simulink library "Library_DataProcessing_v1_1"  (R2021b)
settings: Solver=VariableStepAuto  StartTime=0.0  StopTime=10.0  RelTol=1e-3
libraries: simulink x6, hdlsllib x2
settings Model: Creator=SidharthUrbanMobilit  LastModifiedBy=SiddharthUrbanMobili

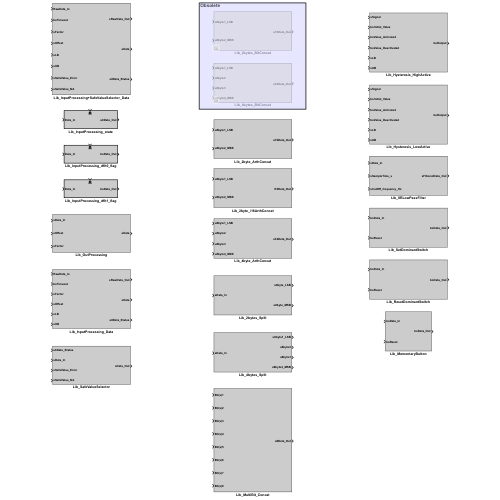
[thumbnail: Simulink's stored preview of the top-level diagram]
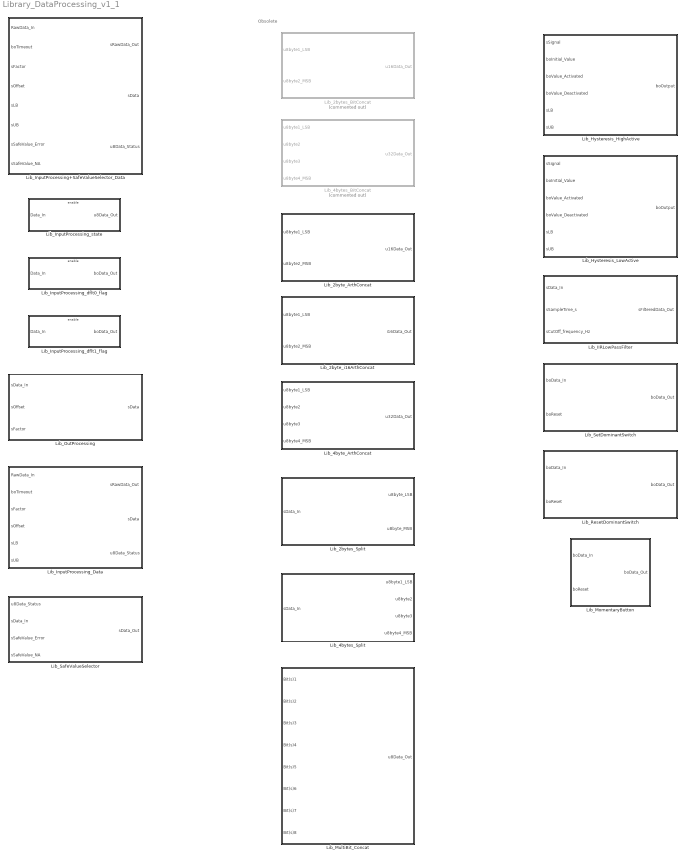
== system Library_DataProcessing_v1_1 ==
  note: Obsolete
  Lib_2byte_ArthConcat : Subsystem
      settings: RTWFcnNameOpts=Use subsystem name  RTWFileNameOpts=Use subsystem name
  Lib_2byte_i16ArthConcat : Subsystem
      settings: RTWFcnNameOpts=Use subsystem name  RTWFileNameOpts=Use subsystem name
  Lib_2bytes_BitConcat : Subsystem  Commented=on
  Lib_2bytes_Split : Subsystem
  Lib_4byte_ArthConcat : Subsystem
      settings: RTWFcnNameOpts=Use subsystem name  RTWFileNameOpts=Use subsystem name
  Lib_4bytes_BitConcat : Subsystem  Commented=on
  Lib_4bytes_Split : Subsystem
  Lib_Hysteresis_HighActive : Subsystem
  Lib_Hysteresis_LowActive : Subsystem
  Lib_IIRLowPassFilter : Subsystem
  Lib_InputProcessing+SafeValueSelector_Data : Subsystem
  Lib_InputProcessing_Data : Subsystem
  Lib_InputProcessing_dflt0_flag : Subsystem
  Lib_InputProcessing_dflt1_flag : Subsystem
  Lib_InputProcessing_state : Subsystem
  Lib_MomentaryButton : Subsystem
  Lib_MultiBit_Concat : Subsystem
      settings: RTWFcnNameOpts=Use subsystem name  RTWFileNameOpts=Use subsystem name
  Lib_OutProcessing : Subsystem
  Lib_ResetDominantSwitch : Subsystem
  Lib_SafeValueSelector : Subsystem
  Lib_SetDominantSwitch : Subsystem

== system Library_DataProcessing_v1_1/Lib_2byte_ArthConcat ==
  u8byte1_LSB : Inport  OutDataTypeStr=uint8
  u8byte2_MSB : Inport  Port=2  OutDataTypeStr=uint8
  Add : Sum  OutDataTypeStr=uint16  RndMeth=Nearest
  Data Type Conversion : DataTypeConversion  OutDataTypeStr=uint16
  Shift Arithmetic : ArithShift  BitShiftNumber=8  BitShiftDirection=Left
  u16Data_Out : Outport
  wires:
  u8byte2_MSB/1 -> Data Type Conversion/1
  Shift Arithmetic/1 -> Add/1
  u8byte1_LSB/1 -> Add/2
  Add/1 -> u16Data_Out/1
  Data Type Conversion/1 -> Shift Arithmetic/1

== system Library_DataProcessing_v1_1/Lib_2byte_i16ArthConcat ==
  u8byte1_LSB : Inport  OutDataTypeStr=uint8
  u8byte2_MSB : Inport  Port=2  OutDataTypeStr=uint8
  Add : Sum  OutDataTypeStr=int16  RndMeth=Nearest
  Data Type Conversion : DataTypeConversion  OutDataTypeStr=int16
  Shift Arithmetic : ArithShift  BitShiftNumber=8  BitShiftDirection=Left
  i16Data_Out : Outport
  wires:
  Data Type Conversion/1 -> Shift Arithmetic/1
  Add/1 -> i16Data_Out/1
  u8byte1_LSB/1 -> Add/2
  Shift Arithmetic/1 -> Add/1
  u8byte2_MSB/1 -> Data Type Conversion/1

== system Library_DataProcessing_v1_1/Lib_2bytes_BitConcat ==
  u8byte1_LSB : Inport  OutDataTypeStr=uint8
  u8byte2_MSB : Inport  Port=2  OutDataTypeStr=uint8
  Bit Concat : hdlsllib/Logic and Bit Operations/Bit Concat  numInputs=2
  Data Type Conversion : DataTypeConversion  OutDataTypeStr=uint16  RndMeth=Nearest
  u16Data_Out : Outport  OutDataTypeStr=uint16
  wires:
  Bit Concat/1 -> Data Type Conversion/1
  Data Type Conversion/1 -> u16Data_Out/1
  u8byte2_MSB/1 -> Bit Concat/1
  u8byte1_LSB/1 -> Bit Concat/2

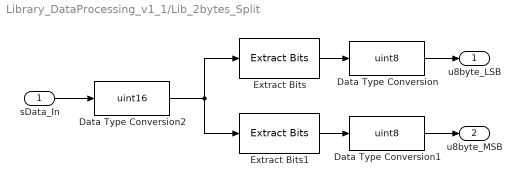
== system Library_DataProcessing_v1_1/Lib_2bytes_Split ==
  sData_In : Inport  OutDataTypeStr=single
  Data Type Conversion : DataTypeConversion  OutDataTypeStr=uint8  RndMeth=Nearest
  Data Type Conversion1 : DataTypeConversion  OutDataTypeStr=uint8  RndMeth=Nearest
  Data Type Conversion2 : DataTypeConversion  OutDataTypeStr=uint16  RndMeth=Nearest
  Extract Bits : simulink/Logic and Bit Operations/Extract Bits  bitsToExtract=Range of bits  numBits=8  bitIdxRange=[0 7]  outScalingMode=Treat bit field as an integer
  Extract Bits1 : simulink/Logic and Bit Operations/Extract Bits  bitsToExtract=Range of bits  numBits=8  bitIdxRange=[8 15]  outScalingMode=Treat bit field as an integer
  u8byte_LSB : Outport
  u8byte_MSB : Outport  Port=2
  wires:
  Extract Bits/1 -> Data Type Conversion/1
  Extract Bits1/1 -> Data Type Conversion1/1
  Data Type Conversion/1 -> u8byte_LSB/1
  Data Type Conversion1/1 -> u8byte_MSB/1
  sData_In/1 -> Data Type Conversion2/1
  Data Type Conversion2/1 -> Extract Bits/1, Extract Bits1/1

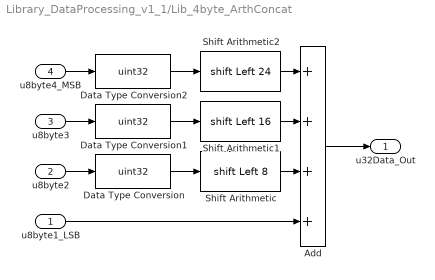
== system Library_DataProcessing_v1_1/Lib_4byte_ArthConcat ==
  u8byte1_LSB : Inport  OutDataTypeStr=uint8
  u8byte2 : Inport  Port=2  OutDataTypeStr=uint8
  u8byte3 : Inport  Port=3  OutDataTypeStr=uint8
  u8byte4_MSB : Inport  Port=4  OutDataTypeStr=uint8
  Add : Sum  Inputs=++++  OutDataTypeStr=uint32  RndMeth=Nearest
  Data Type Conversion : DataTypeConversion  OutDataTypeStr=uint32  RndMeth=Nearest
  Data Type Conversion1 : DataTypeConversion  OutDataTypeStr=uint32  RndMeth=Nearest
  Data Type Conversion2 : DataTypeConversion  OutDataTypeStr=uint32  RndMeth=Nearest
  Shift Arithmetic : ArithShift  BitShiftNumber=8  BitShiftDirection=Left
  Shift Arithmetic1 : ArithShift  BitShiftNumber=16  BitShiftDirection=Left
  Shift Arithmetic2 : ArithShift  BitShiftNumber=24  BitShiftDirection=Left
  u32Data_Out : Outport
  wires:
  Data Type Conversion/1 -> Shift Arithmetic/1
  Add/1 -> u32Data_Out/1
  u8byte2/1 -> Data Type Conversion/1
  Data Type Conversion1/1 -> Shift Arithmetic1/1
  u8byte3/1 -> Data Type Conversion1/1
  Data Type Conversion2/1 -> Shift Arithmetic2/1
  u8byte4_MSB/1 -> Data Type Conversion2/1
  Shift Arithmetic2/1 -> Add/1
  Shift Arithmetic1/1 -> Add/2
  Shift Arithmetic/1 -> Add/3
  u8byte1_LSB/1 -> Add/4

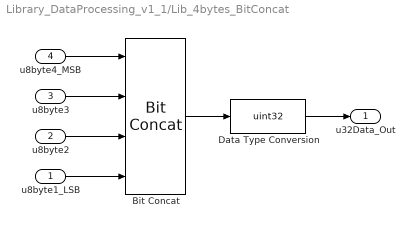
== system Library_DataProcessing_v1_1/Lib_4bytes_BitConcat ==
  u8byte1_LSB : Inport  OutDataTypeStr=uint8
  u8byte2 : Inport  Port=2  OutDataTypeStr=uint8
  u8byte3 : Inport  Port=3  OutDataTypeStr=uint8
  u8byte4_MSB : Inport  Port=4  OutDataTypeStr=uint8
  Bit Concat : hdlsllib/Logic and Bit Operations/Bit Concat  numInputs=4
  Data Type Conversion : DataTypeConversion  OutDataTypeStr=uint32  RndMeth=Nearest
  u32Data_Out : Outport  OutDataTypeStr=uint32
  wires:
  Data Type Conversion/1 -> u32Data_Out/1
  Bit Concat/1 -> Data Type Conversion/1
  u8byte4_MSB/1 -> Bit Concat/1
  u8byte3/1 -> Bit Concat/2
  u8byte2/1 -> Bit Concat/3
  u8byte1_LSB/1 -> Bit Concat/4

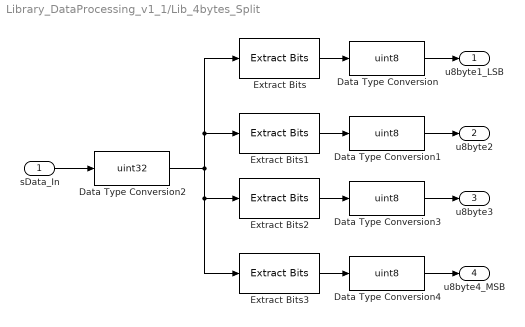
== system Library_DataProcessing_v1_1/Lib_4bytes_Split ==
  sData_In : Inport  OutDataTypeStr=single
  Data Type Conversion{,1,3..4} (4 alike) : DataTypeConversion  OutDataTypeStr=uint8  RndMeth=Nearest
  Data Type Conversion2 : DataTypeConversion  OutDataTypeStr=uint32  RndMeth=Nearest
  Extract Bits : simulink/Logic and Bit Operations/Extract Bits  bitsToExtract=Range of bits  numBits=8  bitIdxRange=[0 7]  outScalingMode=Treat bit field as an integer
  Extract Bits1 : simulink/Logic and Bit Operations/Extract Bits  bitsToExtract=Range of bits  numBits=8  bitIdxRange=[8 15]  outScalingMode=Treat bit field as an integer
  Extract Bits2 : simulink/Logic and Bit Operations/Extract Bits  bitsToExtract=Range of bits  numBits=8  bitIdxRange=[16 23]  outScalingMode=Treat bit field as an integer
  Extract Bits3 : simulink/Logic and Bit Operations/Extract Bits  bitsToExtract=Range of bits  numBits=8  bitIdxRange=[24 31]  outScalingMode=Treat bit field as an integer
  u8byte1_LSB : Outport
  u8byte2 : Outport  Port=2
  u8byte3 : Outport  Port=3
  u8byte4_MSB : Outport  Port=4
  wires:
  Data Type Conversion2/1 -> Extract Bits3/1, Extract Bits2/1, Extract Bits/1, Extract Bits1/1
  sData_In/1 -> Data Type Conversion2/1
  Data Type Conversion1/1 -> u8byte2/1
  Data Type Conversion/1 -> u8byte1_LSB/1
  Extract Bits1/1 -> Data Type Conversion1/1
  Extract Bits/1 -> Data Type Conversion/1
  Extract Bits2/1 -> Data Type Conversion3/1
  Extract Bits3/1 -> Data Type Conversion4/1
  Data Type Conversion3/1 -> u8byte3/1
  Data Type Conversion4/1 -> u8byte4_MSB/1

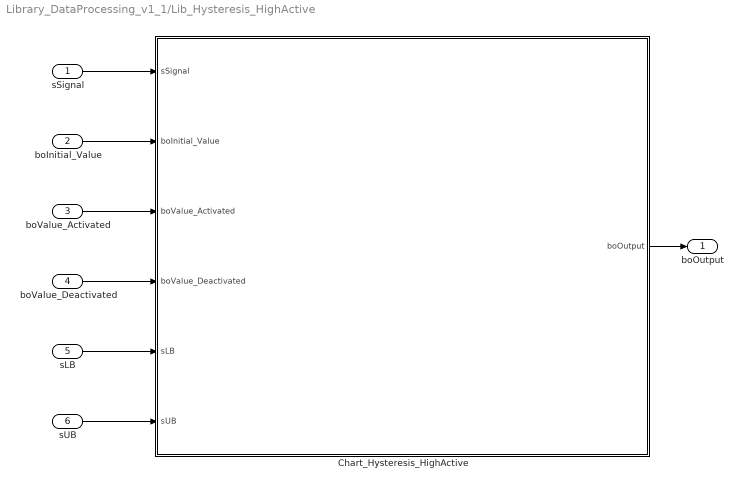
== system Library_DataProcessing_v1_1/Lib_Hysteresis_HighActive ==
  sSignal : Inport  OutDataTypeStr=single
  boInitial_Value : Inport  Port=2  OutDataTypeStr=boolean
  boValue_Activated : Inport  Port=3  OutDataTypeStr=boolean
  boValue_Deactivated : Inport  Port=4  OutDataTypeStr=boolean
  sLB : Inport  Port=5  OutDataTypeStr=single
  sUB : Inport  Port=6  OutDataTypeStr=single
  Chart_Hysteresis_HighActive : Stateflow chart  TreatAsAtomicUnit=on
  boOutput : Outport  OutDataTypeStr=boolean
  wires:
  boInitial_Value/1 -> Chart_Hysteresis_HighActive/2(boInitial_Value)
  boValue_Activated/1 -> Chart_Hysteresis_HighActive/3(boValue_Activated)
  sLB/1 -> Chart_Hysteresis_HighActive/5(sLB)
  sUB/1 -> Chart_Hysteresis_HighActive/6(sUB)
  boValue_Deactivated/1 -> Chart_Hysteresis_HighActive/4(boValue_Deactivated)
  Chart_Hysteresis_HighActive/1(boOutput) -> boOutput/1
  sSignal/1 -> Chart_Hysteresis_HighActive/1(sSignal)

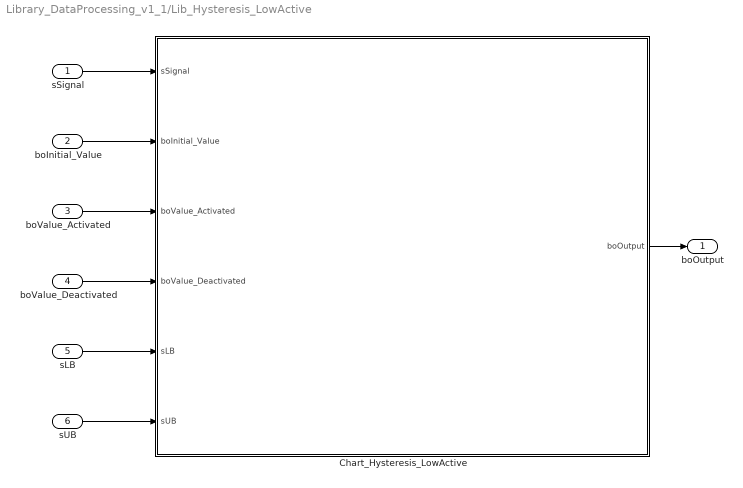
== system Library_DataProcessing_v1_1/Lib_Hysteresis_LowActive ==
  sSignal : Inport  OutDataTypeStr=single
  boInitial_Value : Inport  Port=2  OutDataTypeStr=boolean
  boValue_Activated : Inport  Port=3  OutDataTypeStr=boolean
  boValue_Deactivated : Inport  Port=4  OutDataTypeStr=boolean
  sLB : Inport  Port=5  OutDataTypeStr=single
  sUB : Inport  Port=6  OutDataTypeStr=single
  Chart_Hysteresis_LowActive : Stateflow chart  TreatAsAtomicUnit=on
  boOutput : Outport  OutDataTypeStr=boolean
  wires:
  sSignal/1 -> Chart_Hysteresis_LowActive/1(sSignal)
  Chart_Hysteresis_LowActive/1(boOutput) -> boOutput/1
  boValue_Deactivated/1 -> Chart_Hysteresis_LowActive/4(boValue_Deactivated)
  sUB/1 -> Chart_Hysteresis_LowActive/6(sUB)
  sLB/1 -> Chart_Hysteresis_LowActive/5(sLB)
  boValue_Activated/1 -> Chart_Hysteresis_LowActive/3(boValue_Activated)
  boInitial_Value/1 -> Chart_Hysteresis_LowActive/2(boInitial_Value)

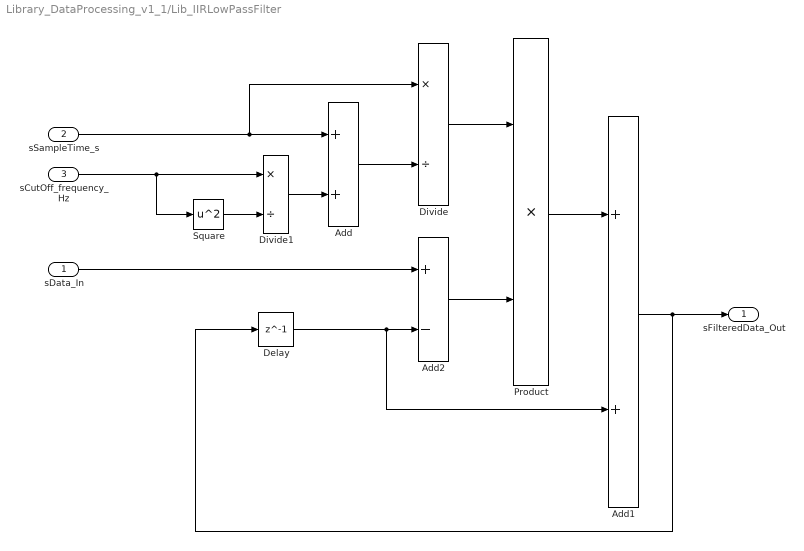
== system Library_DataProcessing_v1_1/Lib_IIRLowPassFilter ==
  sData_In : Inport  OutDataTypeStr=single
  sSampleTime_s : Inport  Port=2  OutDataTypeStr=single
  sCutOff_frequency_Hz : Inport  Port=3  OutDataTypeStr=single
  Add : Sum  OutDataTypeStr=single
  Add1 : Sum  OutDataTypeStr=single
  Add2 : Sum  Inputs=+-  OutDataTypeStr=single
  Delay : Delay  DelayLength=1
  Divide : Product  Inputs=*/  OutDataTypeStr=single
  Divide1 : Product  Inputs=*/  OutDataTypeStr=single
  Product : Product  OutDataTypeStr=single
  Square : Math  Operator=square  SignedPower=on  OutDataTypeStr=single  SaturateOnIntegerOverflow=on
  sFilteredData_Out : Outport  OutDataTypeStr=single  VectorParamsAs1DForOutWhenUnconnected=off
  wires:
  Divide1/1 -> Add/2
  Add2/1 -> Product/2
  sSampleTime_s/1 -> Add/1, Divide/1
  Delay/1 -> Add2/2, Add1/2
  sData_In/1 -> Add2/1
  Add/1 -> Divide/2
  Add1/1 -> Delay/1, sFilteredData_Out/1
  Divide/1 -> Product/1
  Product/1 -> Add1/1
  sCutOff_frequency_Hz/1 -> Square/1, Divide1/1
  Square/1 -> Divide1/2

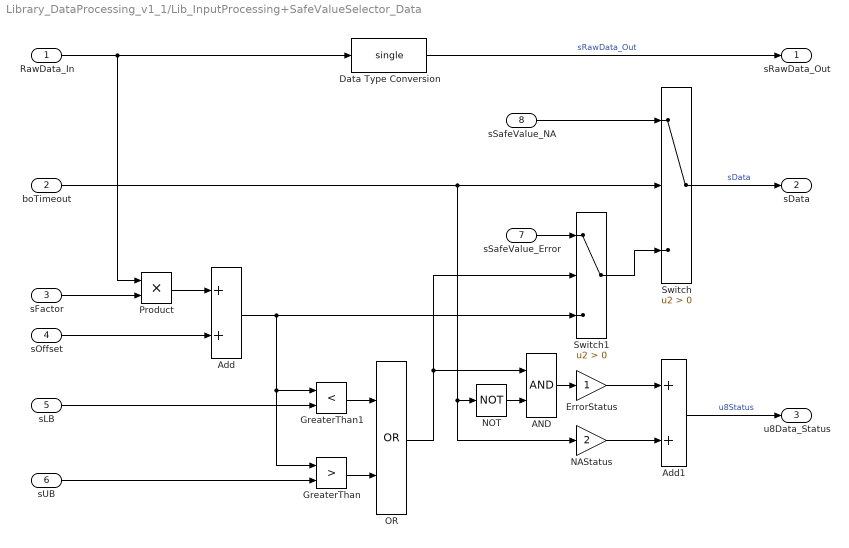
== system Library_DataProcessing_v1_1/Lib_InputProcessing+SafeValueSelector_Data ==
  RawData_In : Inport
  boTimeout : Inport  Port=2  OutDataTypeStr=boolean
  sFactor : Inport  Port=3  OutDataTypeStr=single
  sOffset : Inport  Port=4  OutDataTypeStr=single
  sLB : Inport  Port=5  OutDataTypeStr=single
  sUB : Inport  Port=6  OutDataTypeStr=single
  sSafeValue_Error : Inport  Port=7
  sSafeValue_NA : Inport  Port=8
  AND : Logic  AllPortsSameDT=off  OutDataTypeStr=boolean
  Add : Sum  OutDataTypeStr=single  RndMeth=Nearest
  Add1 : Sum  OutDataTypeStr=uint8  RndMeth=Nearest
  Data Type Conversion : DataTypeConversion  OutDataTypeStr=single  RndMeth=Nearest
  ErrorStatus : Gain  OutDataTypeStr=uint8  RndMeth=Nearest
  GreaterThan : RelationalOperator  Operator=>  OutDataTypeStr=boolean  RndMeth=Simplest
  GreaterThan1 : RelationalOperator  Operator=<  OutDataTypeStr=boolean  RndMeth=Simplest
  NAStatus : Gain  Gain=2  OutDataTypeStr=uint8  RndMeth=Nearest
  NOT : Logic  Operator=NOT  AllPortsSameDT=off  OutDataTypeStr=boolean
  OR : Logic  Operator=OR  AllPortsSameDT=off  OutDataTypeStr=boolean
  Product : Product  OutDataTypeStr=single  RndMeth=Nearest
  Switch : Switch  Criteria=u2 > Threshold  OutDataTypeStr=single  RndMeth=Nearest
  Switch1 : Switch  Criteria=u2 > Threshold  OutDataTypeStr=single  RndMeth=Nearest
  sRawData_Out : Outport  OutDataTypeStr=single
  sData : Outport  Port=2  OutDataTypeStr=single
  u8Data_Status : Outport  Port=3  OutDataTypeStr=uint8
  wires:
  Add/1 -> GreaterThan/1, GreaterThan1/1, Switch1/3
  sOffset/1 -> Add/2
  sSafeValue_Error/1 -> Switch1/1
  Product/1 -> Add/1
  RawData_In/1 -> Product/1, Data Type Conversion/1
  sUB/1 -> GreaterThan/2
  GreaterThan/1 -> OR/2
  Switch/1 -> sData/1  "sData"
  sFactor/1 -> Product/2
  sLB/1 -> GreaterThan1/2
  NAStatus/1 -> Add1/2
  Data Type Conversion/1 -> sRawData_Out/1  "sRawData_Out"
  boTimeout/1 -> NOT/1, NAStatus/1, Switch/2
  ErrorStatus/1 -> Add1/1
  Add1/1 -> u8Data_Status/1  "u8Status"
  Switch1/1 -> Switch/3
  GreaterThan1/1 -> OR/1
  OR/1 -> AND/1, Switch1/2
  NOT/1 -> AND/2
  AND/1 -> ErrorStatus/1
  sSafeValue_NA/1 -> Switch/1

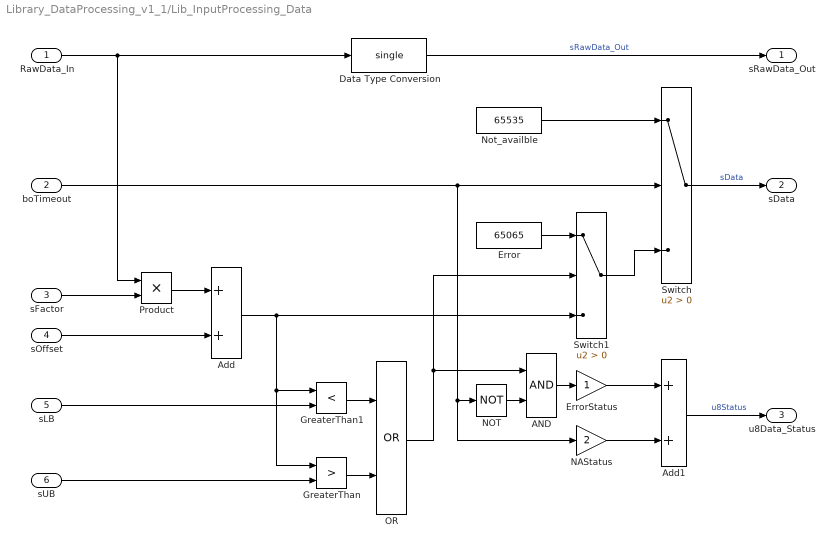
== system Library_DataProcessing_v1_1/Lib_InputProcessing_Data ==
  RawData_In : Inport
  boTimeout : Inport  Port=2  OutDataTypeStr=boolean
  sFactor : Inport  Port=3  OutDataTypeStr=single
  sOffset : Inport  Port=4  OutDataTypeStr=single
  sLB : Inport  Port=5  OutDataTypeStr=single
  sUB : Inport  Port=6  OutDataTypeStr=single
  AND : Logic  AllPortsSameDT=off  OutDataTypeStr=boolean
  Add : Sum  OutDataTypeStr=single  RndMeth=Nearest
  Add1 : Sum  OutDataTypeStr=uint8  RndMeth=Nearest
  Data Type Conversion : DataTypeConversion  OutDataTypeStr=single  RndMeth=Nearest
  Error : Constant  Value=65065  OutDataTypeStr=single
  ErrorStatus : Gain  OutDataTypeStr=uint8  RndMeth=Nearest
  GreaterThan : RelationalOperator  Operator=>  OutDataTypeStr=boolean  RndMeth=Simplest
  GreaterThan1 : RelationalOperator  Operator=<  OutDataTypeStr=boolean  RndMeth=Simplest
  NAStatus : Gain  Gain=2  OutDataTypeStr=uint8  RndMeth=Nearest
  NOT : Logic  Operator=NOT  AllPortsSameDT=off  OutDataTypeStr=boolean
  Not_availble : Constant  Value=65535  OutDataTypeStr=single
  OR : Logic  Operator=OR  AllPortsSameDT=off  OutDataTypeStr=boolean
  Product : Product  OutDataTypeStr=single  RndMeth=Nearest
  Switch : Switch  Criteria=u2 > Threshold  OutDataTypeStr=single  RndMeth=Nearest
  Switch1 : Switch  Criteria=u2 > Threshold  OutDataTypeStr=single  RndMeth=Nearest
  sRawData_Out : Outport  OutDataTypeStr=single
  sData : Outport  Port=2  OutDataTypeStr=single
  u8Data_Status : Outport  Port=3  OutDataTypeStr=uint8
  wires:
  AND/1 -> ErrorStatus/1
  NOT/1 -> AND/2
  OR/1 -> Switch1/2, AND/1
  GreaterThan1/1 -> OR/1
  Switch1/1 -> Switch/3
  Add1/1 -> u8Data_Status/1  "u8Status"
  ErrorStatus/1 -> Add1/1
  boTimeout/1 -> Switch/2, NAStatus/1, NOT/1
  Data Type Conversion/1 -> sRawData_Out/1  "sRawData_Out"
  Not_availble/1 -> Switch/1
  NAStatus/1 -> Add1/2
  sLB/1 -> GreaterThan1/2
  sFactor/1 -> Product/2
  Switch/1 -> sData/1  "sData"
  GreaterThan/1 -> OR/2
  sUB/1 -> GreaterThan/2
  RawData_In/1 -> Data Type Conversion/1, Product/1
  Product/1 -> Add/1
  Error/1 -> Switch1/1
  sOffset/1 -> Add/2
  Add/1 -> Switch1/3, GreaterThan1/1, GreaterThan/1

== system Library_DataProcessing_v1_1/Lib_InputProcessing_dflt0_flag ==
  Data_In : Inport
  Timeout : EnablePort
  Data Type Conversion : DataTypeConversion  OutDataTypeStr=boolean
  boData_Out : Outport  OutDataTypeStr=boolean  OutputWhenDisabled=reset  InitialOutput=[0]
  wires:
  Data_In/1 -> Data Type Conversion/1
  Data Type Conversion/1 -> boData_Out/1

== system Library_DataProcessing_v1_1/Lib_InputProcessing_dflt1_flag ==
  Data_In : Inport  OutDataTypeStr=boolean
  Timeout : EnablePort
  Data Type Conversion : DataTypeConversion  OutDataTypeStr=boolean
  boData_Out : Outport  OutDataTypeStr=boolean  OutputWhenDisabled=reset  InitialOutput=[1]
  wires:
  Data_In/1 -> Data Type Conversion/1
  Data Type Conversion/1 -> boData_Out/1

== system Library_DataProcessing_v1_1/Lib_InputProcessing_state ==
  Data_In : Inport
  Timeout : EnablePort
  Data Type Conversion : DataTypeConversion  OutDataTypeStr=uint8
  u8Data_Out : Outport  OutDataTypeStr=uint8  OutputWhenDisabled=reset  InitialOutput=[0]
  wires:
  Data_In/1 -> Data Type Conversion/1
  Data Type Conversion/1 -> u8Data_Out/1

== system Library_DataProcessing_v1_1/Lib_MomentaryButton ==
  boData_In : Inport  OutDataTypeStr=boolean
  boReset : Inport  Port=2  OutDataTypeStr=boolean
  chart_MomentaryButton : Stateflow chart  TreatAsAtomicUnit=on
  boData_Out : Outport  OutDataTypeStr=boolean
  wires:
  boData_In/1 -> chart_MomentaryButton/1(In)
  chart_MomentaryButton/1(Out) -> boData_Out/1
  boReset/1 -> chart_MomentaryButton/2(reset)

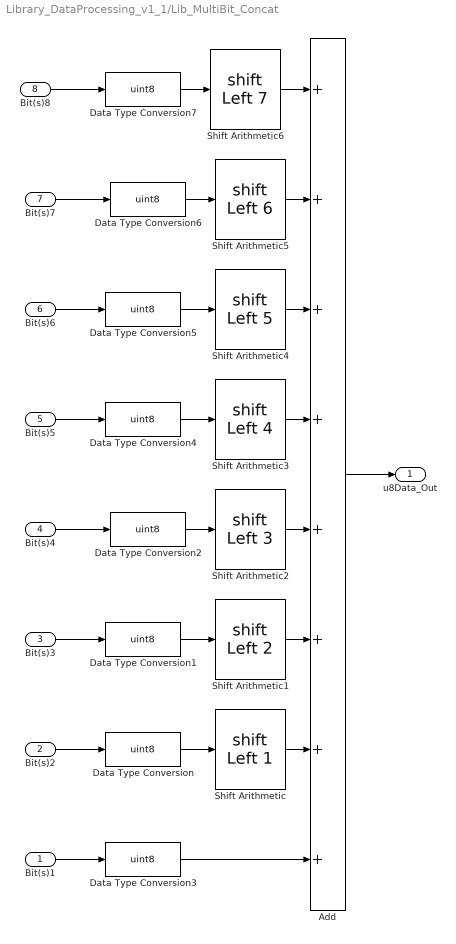
== system Library_DataProcessing_v1_1/Lib_MultiBit_Concat ==
  Bit(s)1 : Inport
  Bit(s)2 : Inport  Port=2
  Bit(s)3 : Inport  Port=3
  Bit(s)4 : Inport  Port=4
  Bit(s)5 : Inport  Port=5
  Bit(s)6 : Inport  Port=6
  Bit(s)7 : Inport  Port=7
  Bit(s)8 : Inport  Port=8
  Add : Sum  Inputs=++++++++  OutDataTypeStr=uint8  RndMeth=Nearest
  Data Type Conversion{,1..7} (8 alike) : DataTypeConversion  OutDataTypeStr=uint8  RndMeth=Nearest
  Shift Arithmetic : ArithShift  BitShiftNumber=1  BitShiftDirection=Left
  Shift Arithmetic1 : ArithShift  BitShiftNumber=2  BitShiftDirection=Left
  Shift Arithmetic2 : ArithShift  BitShiftNumber=3  BitShiftDirection=Left
  Shift Arithmetic3 : ArithShift  BitShiftNumber=4  BitShiftDirection=Left
  Shift Arithmetic4 : ArithShift  BitShiftNumber=5  BitShiftDirection=Left
  Shift Arithmetic5 : ArithShift  BitShiftNumber=6  BitShiftDirection=Left
  Shift Arithmetic6 : ArithShift  BitShiftNumber=7  BitShiftDirection=Left
  u8Data_Out : Outport
  wires:
  Data Type Conversion3/1 -> Add/8
  Data Type Conversion4/1 -> Shift Arithmetic3/1
  Shift Arithmetic/1 -> Add/7
  Bit(s)7/1 -> Data Type Conversion6/1
  Data Type Conversion/1 -> Shift Arithmetic/1
  Shift Arithmetic1/1 -> Add/6
  Shift Arithmetic6/1 -> Add/1
  Bit(s)2/1 -> Data Type Conversion/1
  Data Type Conversion7/1 -> Shift Arithmetic6/1
  Add/1 -> u8Data_Out/1
  Shift Arithmetic3/1 -> Add/4
  Bit(s)5/1 -> Data Type Conversion4/1
  Bit(s)8/1 -> Data Type Conversion7/1
  Shift Arithmetic5/1 -> Add/2
  Shift Arithmetic2/1 -> Add/5
  Bit(s)6/1 -> Data Type Conversion5/1
  Data Type Conversion1/1 -> Shift Arithmetic1/1
  Bit(s)3/1 -> Data Type Conversion1/1
  Bit(s)4/1 -> Data Type Conversion2/1
  Shift Arithmetic4/1 -> Add/3
  Data Type Conversion5/1 -> Shift Arithmetic4/1
  Data Type Conversion6/1 -> Shift Arithmetic5/1
  Bit(s)1/1 -> Data Type Conversion3/1
  Data Type Conversion2/1 -> Shift Arithmetic2/1

== system Library_DataProcessing_v1_1/Lib_OutProcessing ==
  sData_In : Inport  OutDataTypeStr=single
  sOffset : Inport  Port=2  OutDataTypeStr=single
  sFactor : Inport  Port=3  OutDataTypeStr=single
  Add : Sum  Inputs=+-  OutDataTypeStr=single  RndMeth=Nearest
  Divide : Product  Inputs=*/  OutDataTypeStr=single  RndMeth=Nearest
  sData : Outport  OutDataTypeStr=single
  wires:
  sData_In/1 -> Add/1
  sFactor/1 -> Divide/2
  Divide/1 -> sData/1
  sOffset/1 -> Add/2
  Add/1 -> Divide/1

== system Library_DataProcessing_v1_1/Lib_ResetDominantSwitch ==
  boData_In : Inport
  boReset : Inport  Port=2
  Chart_ResetDominantSwitch : Stateflow chart  TreatAsAtomicUnit=on
  boData_Out : Outport
  wires:
  Chart_ResetDominantSwitch/1(boData_Out) -> boData_Out/1
  boReset/1 -> Chart_ResetDominantSwitch/2(boReset)
  boData_In/1 -> Chart_ResetDominantSwitch/1(boData_In)

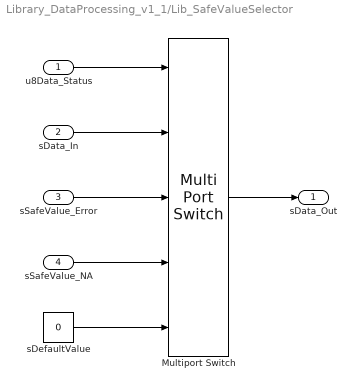
== system Library_DataProcessing_v1_1/Lib_SafeValueSelector ==
  u8Data_Status : Inport
  sData_In : Inport  Port=2
  sSafeValue_Error : Inport  Port=3
  sSafeValue_NA : Inport  Port=4
  Multiport Switch : MultiPortSwitch  DataPortOrder=Zero-based contiguous  DataPortForDefault=Additional data port  DiagnosticForDefault=None  zeroidx=on  OutDataTypeStr=single  RndMeth=Nearest
  sDefaultValue : Constant  Value=0  OutDataTypeStr=single
  sData_Out : Outport
  wires:
  u8Data_Status/1 -> Multiport Switch/1
  sData_In/1 -> Multiport Switch/2
  sSafeValue_Error/1 -> Multiport Switch/3
  sSafeValue_NA/1 -> Multiport Switch/4
  sDefaultValue/1 -> Multiport Switch/5
  Multiport Switch/1 -> sData_Out/1

== system Library_DataProcessing_v1_1/Lib_SetDominantSwitch ==
  boData_In : Inport
  boReset : Inport  Port=2
  Chart_SetDominantSwitch : Stateflow chart  TreatAsAtomicUnit=on
  boData_Out : Outport
  wires:
  boData_In/1 -> Chart_SetDominantSwitch/1(boData_In)
  boReset/1 -> Chart_SetDominantSwitch/2(boReset)
  Chart_SetDominantSwitch/1(boData_Out) -> boData_Out/1

== stateflow chart Library_DataProcessing_v1_1/Lib_Hysteresis_LowActive/Chart_Hysteresis_LowActive ==
  state OFF
    entry:
    boOutput= boInitial_Value;
  state LowValue
    entry:
    boOutput = boValue_Deactivated;
  state HighValue
    entry:
    boOutput = boValue_Activated;
  (default) -> OFF
  OFF -> LowValue [order 1] : [sSignal>sUB]
  OFF -> HighValue [order 2] : [sSignal<sLB]
  HighValue -> LowValue : [sSignal>sUB]
  LowValue -> HighValue : [sSignal<sLB]
  data: sSignal input single; boInitial_Value input boolean; boValue_Activated input boolean; boValue_Deactivated input boolean; boOutput output boolean; sLB input single; sUB input single

== stateflow chart Library_DataProcessing_v1_1/Lib_MomentaryButton/chart_MomentaryButton ==
  state state3
    Out = false;
  state Initial_state
    Out = false;
  state Reset_state
    Out = false;
  state state2
    Out = true;
  state state1
    Out = true;
  (junction 47) -> (junction 48)
  state3 -> (junction 47) [order 2]
  (junction 48) -> Reset_state : [reset == true]
  (default) -> Initial_state
  Initial_state -> Reset_state [order 1] : [reset == true]
  state3 -> Initial_state [order 1] : [In == false]
  Reset_state -> Initial_state : [reset == false]
  state2 -> state3 [order 2] : [In == true]
  Initial_state -> state1 [order 2] : [In == true]
  (junction 41) -> Reset_state : [reset == true]
  state1 -> (junction 41) [order 1]
  state1 -> state2 [order 2] : [In == false]
  (junction 42) -> (junction 41)
  state2 -> (junction 44) [order 1]
  (junction 44) -> (junction 42)
  data: Out output boolean; In input boolean; reset input boolean

== stateflow chart Library_DataProcessing_v1_1/Lib_Hysteresis_HighActive/Chart_Hysteresis_HighActive ==
  state OFF
    entry:
    boOutput= boInitial_Value;
  state LowValue
    entry:
    boOutput = boValue_Deactivated;
  state HighValue
    entry:
    boOutput = boValue_Activated;
  (default) -> OFF
  OFF -> LowValue [order 1] : [sSignal<sLB]
  OFF -> HighValue [order 2] : [sSignal>sUB]
  HighValue -> LowValue : [sSignal<sLB]
  LowValue -> HighValue : [sSignal>sUB]
  data: sSignal input single; boInitial_Value input boolean; boValue_Activated input boolean; boValue_Deactivated input boolean; boOutput output boolean; sLB input single; sUB input single

== stateflow chart Library_DataProcessing_v1_1/Lib_ResetDominantSwitch/Chart_ResetDominantSwitch ==
  state Initial_state
    boData_Out = false;
  state Reset_state
    boData_Out = false;
  state state1
    boData_Out = true;
  state state2
    boData_Out = true;
  (default) -> Initial_state
  Initial_state -> Reset_state [order 2] : [boReset == true]
  Reset_state -> Initial_state : [boReset == false]
  Initial_state -> state1 [order 1] : [boData_In == true]
  (junction 14) -> Reset_state : [boReset == true]
  state1 -> (junction 14) [order 2]
  (junction 16) -> (junction 14)
  state1 -> state2 [order 1] : [boData_In == false]
  state2 -> (junction 16)
  data: boData_In input; boReset input; boData_Out output

== stateflow chart Library_DataProcessing_v1_1/Lib_SetDominantSwitch/Chart_SetDominantSwitch ==
  state Initial_state
    boData_Out = false;
  state Reset_state
    boData_Out = false;
  state state1
    boData_Out = true;
  state state2
    boData_Out = true;
  (default) -> Initial_state
  Reset_state -> Initial_state : [boReset == false]
  Initial_state -> state1 : [boData_In == true]
  state2 -> Reset_state : [boReset == true]
  state1 -> state2 : [boData_In == false]
  data: boData_In input; boReset input; boData_Out output
